simulink model "Modelo_dinamico (2)"  (R2024a)
settings: Solver=VariableStepAuto  StartTime=0.0  StopTime=1000  RelTol=1e-3
settings Model: Creator=alfre
settings RTWCC: GPUComputeCapability=3.5

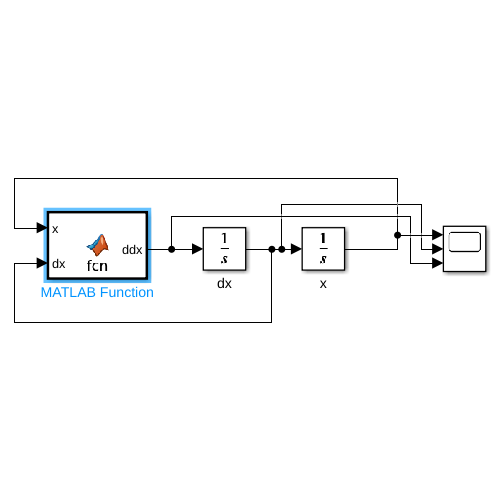
[thumbnail: Simulink's stored preview of the top-level diagram]
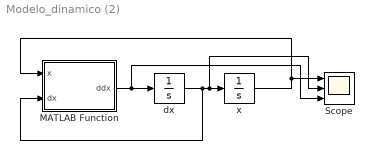
== system Modelo_dinamico (2) ==
  MATLAB Function : MATLAB Function  TreatAsAtomicUnit=on
  Scope : Scope  NumInputPorts=3
  dx : Integrator  ContinuousStateAttributes="\"dx\""
  x : Integrator  ContinuousStateAttributes="\"x\""
  wires:
  MATLAB Function/1(ddx) -> Scope/3, dx/1
  dx/1 -> MATLAB Function/2(dx), Scope/2, x/1
  x/1 -> Scope/1, MATLAB Function/1(x)

== matlab function Modelo_dinamico (2)/MATLAB Function ==
  data: x input; ddx output; dx input
function ddx = fcn(x, dx)
k=0.01;
m=0.75;
g=9.8;
Tau=0;
l = 0.36;
a= l/2;
J = 4/3*m*a^2;
ddx = Tau/J - k*dx/J - m*g*a*cos(x)/J;
